simulink model "crazyflie"  (R2018b)
settings: Solver=FixedStepDiscrete  StartTime=0.0  StopTime=4  FixedStep=0.01  RelTol=1e-3
values from neighbouring files (symbols this model uses):
  K = K0    [Linearization_2.m]
settings Model: PauseTimes=7  Creator=Zrean  LastModifiedBy=Simon
settings OptimizationCC: DefaultParameterBehavior=Inlined  UseDivisionForNetSlopeComputation=on  UseFloatMulNetSlope=on  UseSpecifiedMinMax=on  InlineInvariantSignals=on  PassReuseOutputArgsAs=Individual arguments  ZeroExternalMemoryAtStartup=off  ZeroInternalMemoryAtStartup=off  NoFixptDivByZeroProtection=on  EfficientFloat2IntCast=on  LifeSpan=1
settings DebuggingCC: AlgebraicLoopMsg=error  ParameterTunabilityLossMsg=error
settings HardwareCC: ProdBitPerPointer=32  ProdBitPerSizeT=32  ProdBitPerPtrDiffT=32  ProdLargestAtomicInteger=Long  ProdLargestAtomicFloat=Double  ProdWordSize=32  ProdHWDeviceType=ARM Compatible->ARM Cortex
settings SFSimCC: SimUseLocalCustomCode=off  MATLABDynamicMemAlloc=off
settings RTWCC: SystemTargetFile=ert.tlc  GenCodeOnly=on  TemplateMakefile=ert_default_tmf  GenerateReport=on  RTWUseLocalCustomCode=off  BuildConfiguration=Faster Runs  IncludeHyperlinkInReport=on  LaunchReport=on  GenerateTraceInfo=on  GenerateTraceReport=on  GenerateTraceReportSl=on  GenerateTraceReportSf=on  GenerateTraceReportEml=on  GenerateCodeMetricsReport=on
settings CodeAppCC: ForceParamTrailComments=on  IgnoreCustomStorageClasses=off  OperatorAnnotations=on  SimulinkDataObjDesc=on  SFDataObjDesc=on  MATLABFcnDesc=on  CustomSymbolStrGlobalVar=rt$N$M  CustomSymbolStrType=$N$M  CustomSymbolStrFcn=$N$M$F  CustomSymbolStrMacro=$N$M  InsertBlockDesc=on  StateflowObjectComments=on  MATLABSourceComments=on
settings ERTTargetCC: TargetLangStandard=C99 (ISO)  MultiwordLength=2048  CombineSignalStateStructs=on  SuppressErrorStatus=on  SupportAbsoluteTime=off  SupportNonFinite=off  SupportComplex=off  InlinedParameterPlacement=NonHierarchical  ERTCustomFileTemplate=crazyflie_wrapper.tlc  ERTFilePackagingFormat=CompactWithDataFile
settings SimscapeCC: SimscapeNormalizeSystem=off

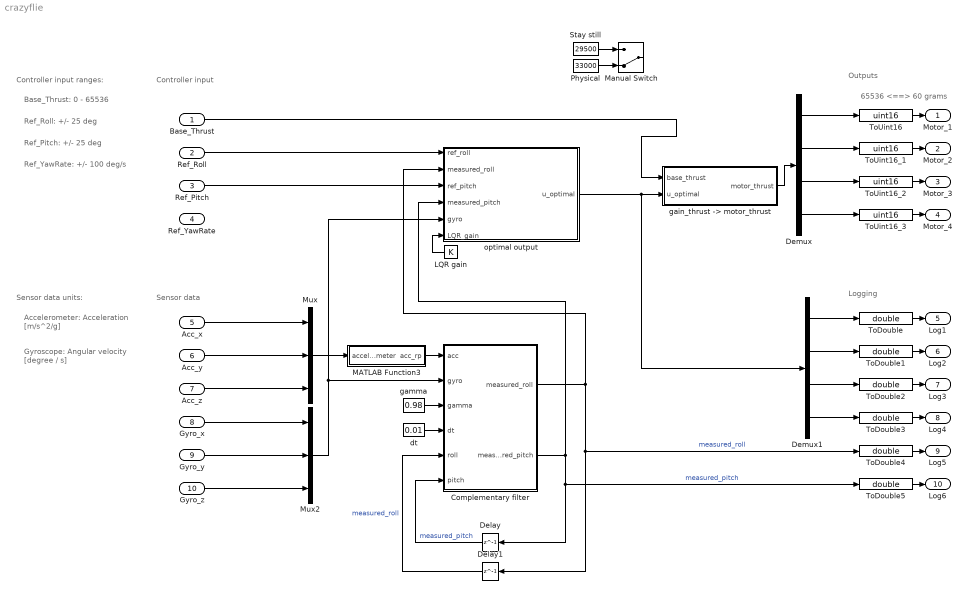
== system crazyflie ==
  note: 65536 <==> 60 grams
  note: Logging
  note: Outputs
  note: Sensor data
  note: Controller input
  note: Ref_Roll: +/- 25 deg
  note: Base_Thrust: 0 - 65536
  note: Ref_Pitch: +/- 25 deg
  note: Ref_YawRate: +/- 100 deg/s
  note: Controller input ranges:
  note: Gyroscope:
      | Angular velocity [degree / s]
  note: Accelerometer:
      | Acceleration [m/s^2/g]
  note: Sensor data units:
  Base_Thrust : Inport  OutDataTypeStr=double
  Ref_Roll : Inport  Port=2  OutDataTypeStr=double
  Ref_Pitch : Inport  Port=3  OutDataTypeStr=double
  Ref_YawRate : Inport  Port=4  OutDataTypeStr=double
  Acc_x : Inport  Port=5  OutDataTypeStr=double  PortDimensions=1
  Acc_y : Inport  Port=6  OutDataTypeStr=double  PortDimensions=1
  Acc_z : Inport  Port=7  OutDataTypeStr=double  PortDimensions=1
  Gyro_x : Inport  Port=8  OutDataTypeStr=double  PortDimensions=1
  Gyro_y : Inport  Port=9  OutDataTypeStr=double  PortDimensions=1
  Gyro_z : Inport  Port=10  OutDataTypeStr=double  PortDimensions=1
  Complementary filter : MATLAB Function  TreatAsAtomicUnit=on
  Delay : Delay  DelayLength=1
  Delay1 : Delay  DelayLength=1
  Demux : Demux
  Demux1 : Demux
  LQR gain : Constant  Value=K  VectorParams1D=off
  MATLAB Function3 : MATLAB Function  TreatAsAtomicUnit=on
  Manual Switch : ManualSwitch  CurrentSetting=0
  Mux : Mux  Inputs=3
  Mux2 : Mux  Inputs=3
  Physical : Constant  Value=33000
  Stay still : Constant  Value=29500
  ToDouble{,1..5} (6 alike) : DataTypeConversion  OutDataTypeStr=double  SaturateOnIntegerOverflow=on
  ToUint16 : DataTypeConversion  OutDataTypeStr=uint16  SaturateOnIntegerOverflow=on
  ToUint16_1 : DataTypeConversion  OutDataTypeStr=uint16  SaturateOnIntegerOverflow=on
  ToUint16_2 : DataTypeConversion  OutDataTypeStr=uint16  SaturateOnIntegerOverflow=on
  ToUint16_3 : DataTypeConversion  OutDataTypeStr=uint16  SaturateOnIntegerOverflow=on
  dt : Constant  Value=0.01
  "gain_thrust -> motor_thrust" : MATLAB Function  TreatAsAtomicUnit=on
  gamma : Constant  Value=0.98
  optimal output : MATLAB Function  TreatAsAtomicUnit=on
  Motor_1 : Outport  OutDataTypeStr=uint16  LockScale=on
  Motor_2 : Outport  Port=2  OutDataTypeStr=uint16  LockScale=on
  Motor_3 : Outport  Port=3  OutDataTypeStr=uint16  LockScale=on
  Motor_4 : Outport  Port=4  OutDataTypeStr=uint16  LockScale=on
  Log1 : Outport  Port=5  OutDataTypeStr=double
  Log2 : Outport  Port=6  OutDataTypeStr=double
  Log3 : Outport  Port=7  OutDataTypeStr=double
  Log4 : Outport  Port=8  OutDataTypeStr=double
  Log5 : Outport  Port=9  OutDataTypeStr=double
  Log6 : Outport  Port=10  OutDataTypeStr=double
  wires:
  ToUint16/1 -> Motor_1/1
  ToUint16_1/1 -> Motor_2/1
  ToUint16_2/1 -> Motor_3/1
  ToUint16_3/1 -> Motor_4/1
  ToDouble/1 -> Log1/1
  ToDouble1/1 -> Log2/1
  ToDouble2/1 -> Log3/1
  ToDouble3/1 -> Log4/1
  ToDouble4/1 -> Log5/1
  ToDouble5/1 -> Log6/1
  Acc_z/1 -> Mux/3
  Acc_y/1 -> Mux/2
  Acc_x/1 -> Mux/1
  Gyro_y/1 -> Mux2/2
  Gyro_x/1 -> Mux2/1
  Mux/1 -> MATLAB Function3/1(accelerometer)
  gamma/1 -> Complementary filter/3(gamma)
  dt/1 -> Complementary filter/4(dt)
  Complementary filter/1(measured_roll) -> optimal output/2(measured_roll), Delay1/1, ToDouble4/1  "measured_roll"
  Complementary filter/2(measured_pitch) -> ToDouble5/1, Delay/1, optimal output/4(measured_pitch)  "measured_pitch"
  Demux/4 -> ToUint16_3/1
  Demux/3 -> ToUint16_2/1
  Demux/2 -> ToUint16_1/1
  Demux/1 -> ToUint16/1
  "gain_thrust -> motor_thrust"/1(motor_thrust) -> Demux/1
  Demux1/1 -> ToDouble/1
  Demux1/2 -> ToDouble1/1
  Demux1/3 -> ToDouble2/1
  Demux1/4 -> ToDouble3/1
  Gyro_z/1 -> Mux2/3
  LQR gain/1 -> optimal output/6(LQR_gain)
  Ref_Roll/1 -> optimal output/1(ref_roll)
  Ref_Pitch/1 -> optimal output/3(ref_pitch)
  Mux2/1 -> Complementary filter/2(gyro), optimal output/5(gyro)
  Delay/1 -> Complementary filter/6(pitch)  "measured_pitch"
  Delay1/1 -> Complementary filter/5(roll)  "measured_roll"
  MATLAB Function3/1(acc_rp) -> Complementary filter/1(acc)
  optimal output/1(u_optimal) -> Demux1/1, "gain_thrust -> motor_thrust"/2(u_optimal)
  Base_Thrust/1 -> "gain_thrust -> motor_thrust"/1(base_thrust)
  Stay still/1 -> Manual Switch/1
  Physical/1 -> Manual Switch/2

== matlab function crazyflie/Complementary filter ==
  data: acc input; measured_roll output; gyro input; gamma input; dt input; roll input; pitch input; measured_pitch output
function [measured_roll, measured_pitch] = fcn(acc,gyro,gamma,dt,roll, pitch)
	if nargin < 5
		roll = 0;
		pitch = 0;
	end
	measured_roll = (gamma)*(roll+gyro(1)*dt)+(1-gamma)*acc(1);
	measured_pitch = (gamma)*(pitch+gyro(2)*dt)+(1-gamma)*acc(2);
end

== matlab function crazyflie/optimal output ==
  data: ref_roll input; measured_roll input; ref_pitch input; u_optimal output; measured_pitch input; gyro input; LQR_gain input
function u_optimal = fcn(ref_roll, measured_roll, ref_pitch, measured_pitch, gyro, LQR_gain)

u = [
	ref_roll-measured_roll;
	ref_pitch-measured_pitch;
	0-gyro(1);
	0-gyro(2);
	0-gyro(3)
	];
thrust_conversion= 1/(0.06/4*9.81/65536);
angle_conversion = pi/180;
K = LQR_gain;
% K = [-0.0130516411025351 -0.0134352368017384 -0.0107871368960590 -0.0111041774433157 -0.00499998563150369;-0.0130516411029438 0.0134352368019400 -0.0107871368966255 0.0111041774440371 0.00499998563150644;0.0130516411030164 0.0134352368022339 0.0107871368964568 0.0111041774437252 -0.00499998563150448;0.0130516411026696 -0.0134352368020933 0.0107871368958907 -0.0111041774430040 0.00499998563150769]
u_optimal = K*u.*thrust_conversion*angle_conversion;

== matlab function crazyflie/MATLAB Function3 ==
  data: accelerometer input; acc_rp output
function acc_rp = fcn(accelerometer)
	acc_x=accelerometer(1);
	acc_y=accelerometer(2);
	acc_z=accelerometer(3);

	if acc_x == 0 && acc_y == 0 && acc_z == 0
		roll = 0;
		pitch = 0;
		acc_rp=[roll;pitch];
		return
	end

	y_n=acc_y/sqrt(acc_x^2+acc_y^2+acc_z^2);
	z_n=acc_z/sqrt(acc_x^2+acc_y^2+acc_z^2);
	x_n=acc_x/sqrt(acc_x^2+acc_y^2+acc_z^2);

	roll=atan2d(y_n,z_n);
	pitch = atan2d(-x_n,sqrt(y_n^2+z_n^2));

	acc_rp=[roll;pitch];

end

== matlab function crazyflie/gain_thrust -> motor_thrust ==
  data: base_thrust input; motor_thrust output; u_optimal input
function motor_thrust = fcn(base_thrust, u_optimal)
    motor_thrust = u_optimal+base_thrust;
    
    for i = 1:length(motor_thrust)
        motor_thrust(i) = max([0,motor_thrust(i)]);
        motor_thrust(i) = min([65536,motor_thrust(i)]);
    end
end
